simulink model "Sim_Model_2ndODE_ex5"  (R2012b)
settings: Solver=ode45  StartTime=pi/3  StopTime=5*pi  RelTol=1e-3
settings Model: Creator=David  LastModifiedBy=David
settings DataIOCC: SignalLoggingSaveFormat=ModelDataLogs
settings DebuggingCC: FcnCallInpInsideContextMsg=UseLocalSettings
settings GRTTargetCC: CombineOutputUpdateFcns=off  GRTInterface=on

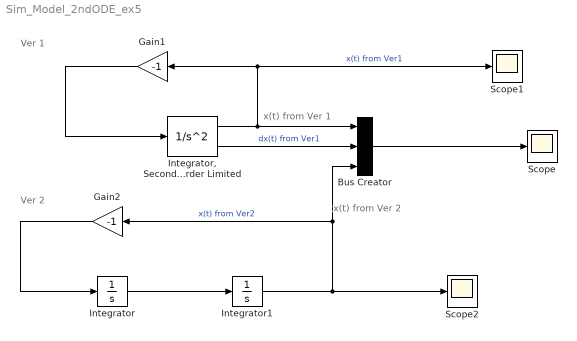
== system Sim_Model_2ndODE_ex5 ==
  note: x(t) from Ver 2
  note: x(t) from Ver 1
  note: Ver 2
  note: Ver 1
  Bus Creator : BusCreator  Inputs=3
  Gain1 : Gain  Gain=-1
  Gain2 : Gain  Gain=-1
  Integrator : Integrator  InitialCondition=-4
  "Integrator, Second-Order Limited" : SecondOrderIntegrator  ICX=2  UpperLimitX=1  LowerLimitX=0  ICDXDT=-4
  Integrator1 : Integrator  InitialCondition=2
  Scope : Scope
      settings: ShowLegends=on
  Scope1 : Scope
  Scope2 : Scope
      settings: SaveName=ScopeData2
  wires:
  "Integrator, Second-Order Limited"/1 -> Bus Creator/1, Scope1/1, Gain1/1  "x(t) from Ver1"
  Bus Creator/1 -> Scope/1
  Integrator/1 -> Integrator1/1
  Integrator1/1 -> Scope2/1, Bus Creator/3, Gain2/1  "x(t) from Ver2"
  "Integrator, Second-Order Limited"/2 -> Bus Creator/2  "dx(t) from Ver1"
  Gain1/1 -> "Integrator, Second-Order Limited"/1
  Gain2/1 -> Integrator/1
